simulink model "Robot_Sim_Model"  (R2021a)
settings: Solver=VariableStepAuto  StartTime=0.0  StopTime=10.0  RelTol=1e-3
values from neighbouring files (symbols this model uses):
  Kc = 4    [Robot_model_param.m]
  Km = 7    [Robot_model_param.m]
  SqWaveFreq = 1/6    (= 0.166666666667)    [Robot_model_param.m]
  ThDotRef = 210    [Robot_model_param.m]
  Tm = 0.4    [Robot_model_param.m]
  Ts = 0.005    [Robot_model_param.m]
  Vm = 30    [Robot_model_param.m]
undefined symbols (not defined in the file or in its folder): COLden, COLnum, DiscIntNeverNeededParam
libraries: simulink x1
settings Model: Creator=asaberi  LastModifiedBy=ZYT
settings SolverCC: AlgebraicLoopSolver=TrustRegion
settings DebuggingCC: SFMachineParentedDataDiag=warning

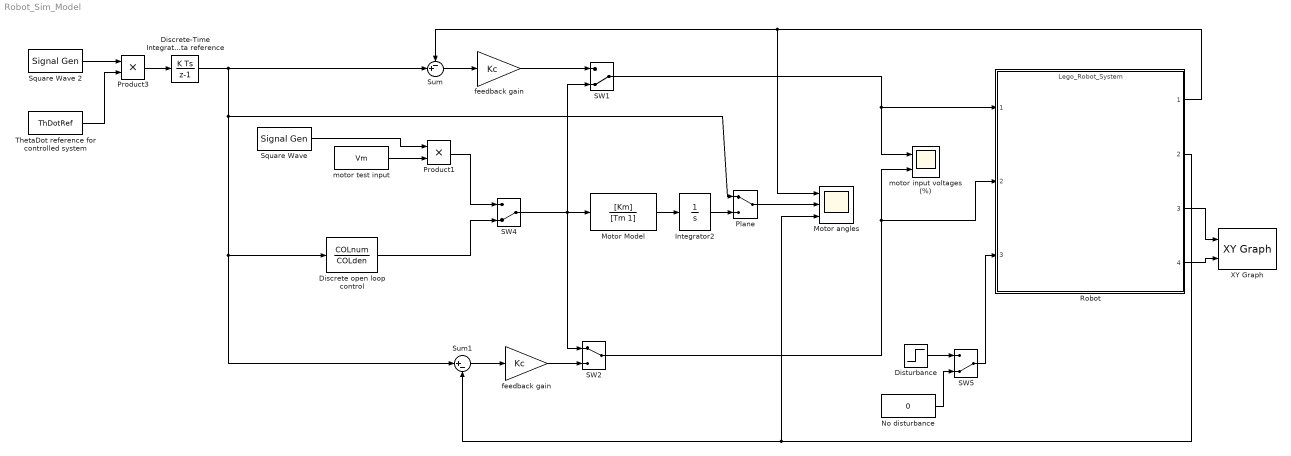
== system Robot_Sim_Model ==
  Discrete open loop control : DiscreteTransferFcn  Numerator=COLnum  Denominator=COLden
  Discrete-Time Integrator to convert ThetaDot reference to a Theta reference : DiscreteIntegrator  SampleTime=Ts  ICPrevOutput=DiscIntNeverNeededParam  ICPrevScaledInput=DiscIntNeverNeededParam
  Disturbance : Step  Time=5  After=-20
  Integrator2 : Integrator
  Motor Model : TransferFcn  Numerator=[Km]  Denominator=[Tm 1]
  Motor angles : Scope  NumInputPorts=3
  No disturbance : Constant  Value=0  SampleTime=-1
  "Plane " : ManualSwitch
  Product1 : Product
  Product3 : Product
  Robot : ModelReference  ModelNameDialog=Lego_Robot_System.slxp  ModelReferenceVersion=1.4  CopyOfModelProtected=on
  SW1 : ManualSwitch  CurrentSetting=0
  SW2 : ManualSwitch
  SW4 : ManualSwitch  CurrentSetting=0
  SW5 : ManualSwitch  CurrentSetting=0
  "Square Wave " : SignalGenerator  WaveForm=square  Frequency=SqWaveFreq
  Square Wave 2 : SignalGenerator  WaveForm=square  Frequency=SqWaveFreq
  Sum : Sum  Inputs=-+|
  Sum1 : Sum  Inputs=|+-
  ThetaDot reference for controlled system : Constant  Value=ThDotRef
  XY Graph : simulink/Sinks/XY Graph  xmin=-15  xmax=1  ymin=-1  ymax=1  st=-1
  feedback gain : Gain  Gain=Kc
  "feedback gain " : Gain  Gain=Kc
  "motor input voltages (%) " : Scope  NumInputPorts=2
  motor test input : Constant  Value=Vm
  wires:
  Robot/1 -> Motor angles/1, Sum/1
  Robot/3 -> XY Graph/1
  Robot/2 -> Sum1/2, Motor angles/3
  SW5/1 -> Robot/3
  SW2/1 -> Robot/2, "motor input voltages (%) "/2
  Product3/1 -> Discrete-Time Integrator to convert ThetaDot reference to a Theta reference/1
  ThetaDot reference for controlled system/1 -> Product3/2
  Robot/4 -> XY Graph/2
  motor test input/1 -> Product1/2
  Motor Model/1 -> Integrator2/1
  Disturbance/1 -> SW5/1
  Product1/1 -> SW4/1
  No disturbance/1 -> SW5/2
  "Square Wave "/1 -> Product1/1
  Integrator2/1 -> "Plane "/2
  "feedback gain "/1 -> SW2/2
  Sum1/1 -> "feedback gain "/1
  Sum/1 -> feedback gain/1
  Square Wave 2/1 -> Product3/1
  SW1/1 -> Robot/1, "motor input voltages (%) "/1
  feedback gain/1 -> SW1/1
  Discrete-Time Integrator to convert ThetaDot reference to a Theta reference/1 -> Discrete open loop control/1, Sum1/1, "Plane "/1, Sum/2
  SW4/1 -> SW2/1, Motor Model/1, SW1/2
  "Plane "/1 -> Motor angles/2
  Discrete open loop control/1 -> SW4/2
